simulink model "SF5_5_9_jc0655"  (R2016b)
settings: Solver=VariableStepAuto  StartTime=0.0  StopTime=10.0  RelTol=1e-3  EnableMultiTasking=on
settings Model: Creator=amyyang  LastModifiedBy=amyyang
settings DataIOCC: LimitDataPoints=on
settings OptimizationCC: LifeSpan=inf
settings DebuggingCC: AllowSymbolicDim=off  SFUnexpectedBacktrackingDiag=warning  SFNoUnconditionalDefaultTransitionDiag=warning  SFExecutionAtInitializationDiag=none
settings ModelReferenceCC: PropagateSignalLabelsOutOfModel=off
settings GRTTargetCC: TargetLangStandard=C89/C90 (ANSI)
settings ConfigComp: CovMetricSettings=dw  CovHtmlReporting=on  CovSaveCumulativeToWorkspaceVar=on  CovSaveSingleToWorkspaceVar=on  CovExternalEMLEnable=off

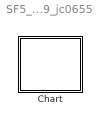
== system SF5_5_9_jc0655 ==
  Chart : Stateflow chart  TreatAsAtomicUnit=on

== stateflow chart SF5_5_9_jc0655/Chart ==
  state Correct [parallel]
    settings: executionOrder=1
    state OFF
    state ON
    (default) -> OFF
    OFF -> ON : [ONflag]
    ON -> OFF : [ ~ONflag]
  state Incorrect [parallel]
    settings: executionOrder=2
    state OFF1
    state ON1
    (default) -> OFF1
    OFF1 -> ON1 : [ONflag ~= 0]
    ON1 -> OFF1 : [ ONflag == 0]
  note: [!ONflag]
